simulink model "MSD_simulation"  (R2022b)
settings: Solver=FixedStepAuto  StartTime=0.0  StopTime=60  FixedStep=0.001  RelTol=1e-6
PreLoadFcn:
  | % Initial Condition
  | m = 1;
  | b = 0.3;
  | k = 2;
  | 
  | % State-Space
  | A = [0 1; -k/m -b/m];
  | B = [0; 1/m];
  | C = [1 0];
  | D = 0;
  | 
  | % Transfer function
  | [Num, Den] = ss2tf(A,B,C,D);
undefined symbols (not defined in the file or in its folder): Den, Num
settings Model: Creator=user  LastModifiedBy=user

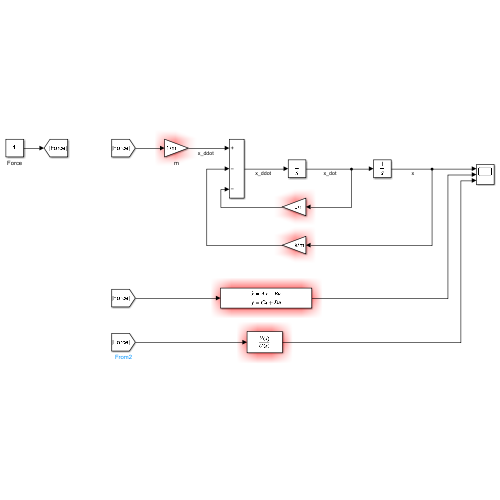
[thumbnail: Simulink's stored preview of the top-level diagram]
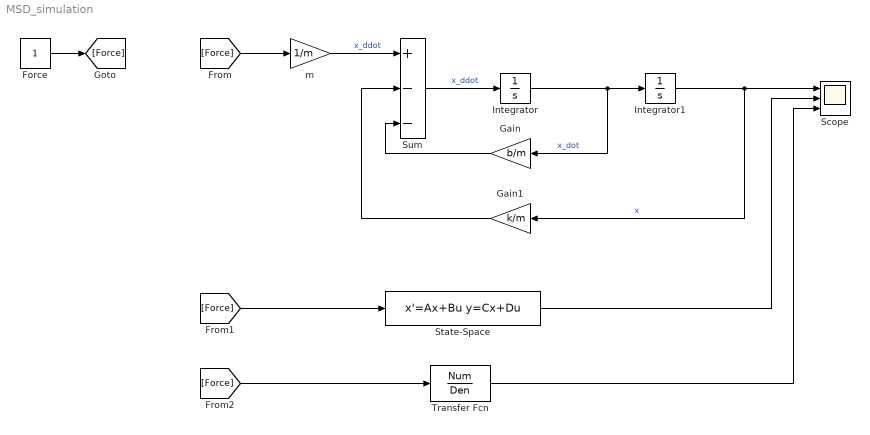
== system MSD_simulation ==
  Force : Constant
  Gain : Gain  Gain=b/m
  Gain1 : Gain  Gain=k/m
  Integrator : Integrator
  Integrator1 : Integrator
  Scope : Scope  NumInputPorts=3
  State-Space : StateSpace  A=A  B=B  C=C  D=D  InitialCondition=0
  Sum : Sum  Inputs=+--
  Transfer Fcn : TransferFcn  Numerator=Num  Denominator=Den
  m : Gain  Gain=1/m
  wires:
  Integrator/1 -> Gain/1, Integrator1/1  "x_dot"
  Integrator1/1 -> Scope/1, Gain1/1  "x"
  m/1 -> Sum/1  "x_ddot"
  Sum/1 -> Integrator/1  "x_ddot"
  Gain/1 -> Sum/3
  Gain1/1 -> Sum/2
  Force/1 -> [Force]
  [Force] -> m/1
  [Force] -> State-Space/1
  [Force] -> Transfer Fcn/1
  State-Space/1 -> Scope/2
  Transfer Fcn/1 -> Scope/3
